simulink model "TX"  (R2024b)
settings: Solver=VariableStepAuto  StartTime=0.0  StopTime=10.0  RelTol=1e-3
settings Model: Creator=User  LastModifiedBy=User

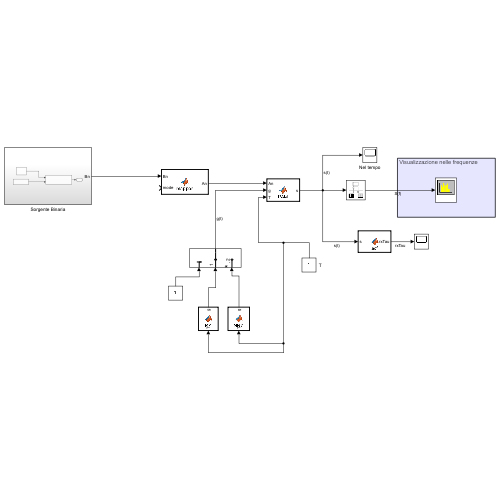
[thumbnail: Simulink's stored preview of the top-level diagram]
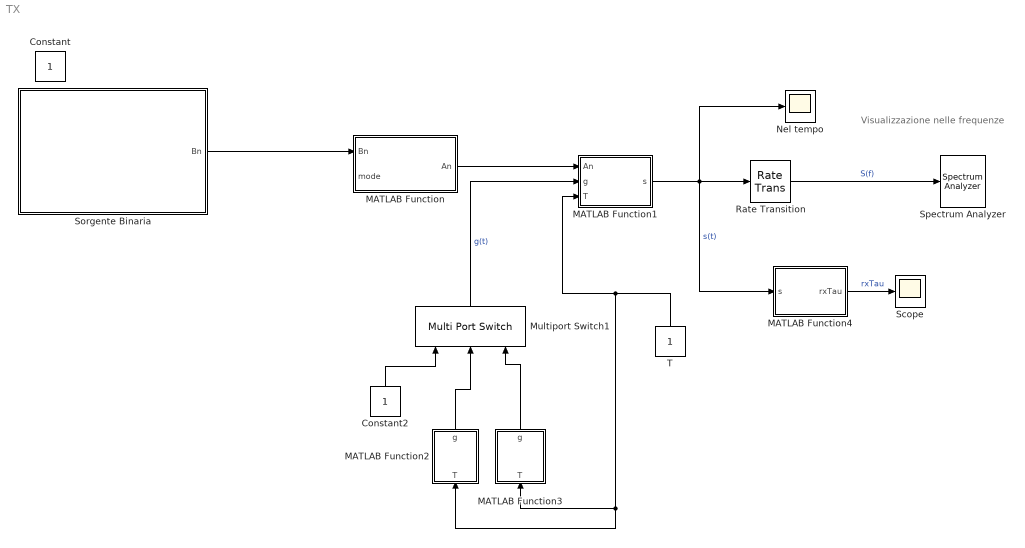
== system TX ==
  note: Visualizzazione nelle frequenze
  Constant2 : Constant
  MATLAB Function : MATLAB Function  TreatAsAtomicUnit=on
  MATLAB Function1 : MATLAB Function  TreatAsAtomicUnit=on
  MATLAB Function2 : MATLAB Function  TreatAsAtomicUnit=on
  MATLAB Function3 : MATLAB Function  TreatAsAtomicUnit=on
  MATLAB Function4 : MATLAB Function  TreatAsAtomicUnit=on
  Multiport Switch1 : MultiPortSwitch  Inputs=2  SaturateOnIntegerOverflow=off  InputSameDT=off
  Nel tempo : Scope
  Rate Transition : RateTransition
  Scope : Scope
  Sorgente Binaria : Subsystem
  Spectrum Analyzer : SpectrumAnalyzer  Method=Welch  PlotAsTwoSidedSpectrum=off  AveragingMethod=Exponential
  T : Constant
  Constant : Constant  IOType=siggen
  wires:
  Sorgente Binaria/1(Bn) -> MATLAB Function/1(Bn)
  MATLAB Function/1(An) -> MATLAB Function1/1(An)
  MATLAB Function1/1(s) -> MATLAB Function4/1(s), Nel tempo/1, Rate Transition/1  "s(t)"
  Rate Transition/1 -> Spectrum Analyzer/1  "S(f)"
  T/1 -> MATLAB Function2/1(T), MATLAB Function3/1(T), MATLAB Function1/3(T)
  Multiport Switch1/1 -> MATLAB Function1/2(g)  "g(t)"
  MATLAB Function2/1(g) -> Multiport Switch1/2
  MATLAB Function3/1(g) -> Multiport Switch1/3
  Constant2/1 -> Multiport Switch1/1
  MATLAB Function4/1(rxTau) -> Scope/1  "rxTau"

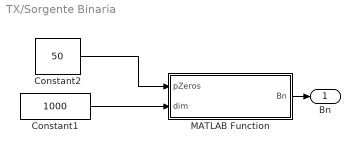
== system TX/Sorgente Binaria ==
  Constant1 : Constant  Value=1000
  Constant2 : Constant  Value=50
  MATLAB Function : MATLAB Function  TreatAsAtomicUnit=on
  Bn : Outport
  wires:
  Constant1/1 -> MATLAB Function/2(dim)
  Constant2/1 -> MATLAB Function/1(pZeros)
  MATLAB Function/1(Bn) -> Bn/1

== matlab function TX/Sorgente Binaria/MATLAB Function ==
  data: pZeros input; Bn output; dim input
function Bn = sorgenteBinaria(pZeros, dim)
    Bn = rand(1,dim) > (pZeros/100);
end

== matlab function TX/MATLAB Function1 ==
  data: An input; s output; g input; T input
function s = PAM(An, g, T)

end

== matlab function TX/MATLAB Function2 ==
  data: T input; g output
function g = RZ(T)

end

== matlab function TX/MATLAB Function3 ==
  data: T input; g output
function g = NRZ(T)

y = u;

== matlab function TX/MATLAB Function4 ==
  data: s input; rxTau output
function rxTau = acf(s)
end

== matlab function TX/MATLAB Function ==
  data: Bn input; An output; mode input
function An = mapper(Bn, mode)
    switch mode
        % Nessuna codifica
        case 1
            An = Bn;
        % Codifica bipolare
        case 2
            Bn(Bn == 0) = -1;
            An = Bn;
    end
end
